simulink model "bit_sum8"  (R2014a)
settings: Solver=FixedStepDiscrete  StartTime=0.0  StopTime=10.0  RelTol=1e-3
InitFcn:
  | %% DSPBuilder Start
  | alt_dspbuilder_update_model(bdroot)
  | %% DSPBuilder End
model workspace (MAT data in the model file):
  Fs = 48000
libraries: simulink x16
settings Model: Creator=User  LastModifiedBy=User
settings DataIOCC: SaveOutput=off  SaveTime=off
settings OptimizationCC: InlineParams=on

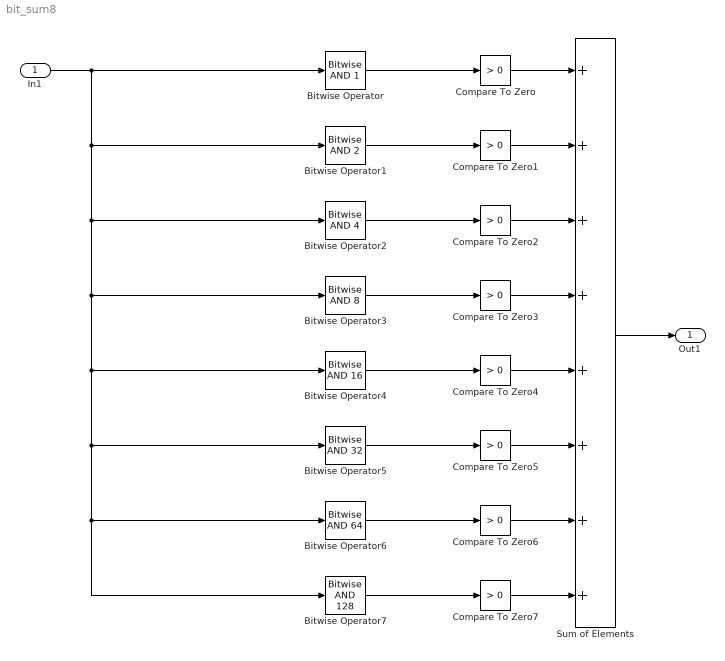
== system bit_sum8 ==
  In1 : Inport  OutDataTypeStr=uint8  PortDimensions=1
  Bitwise Operator : simulink/Logic and Bit Operations/Bitwise Operator  logicop=AND  UseBitMask=on  BitMask=1  BitMaskRealWorld=Stored Integer
  Bitwise Operator1 : simulink/Logic and Bit Operations/Bitwise Operator  logicop=AND  UseBitMask=on  BitMask=2  BitMaskRealWorld=Stored Integer
  Bitwise Operator2 : simulink/Logic and Bit Operations/Bitwise Operator  logicop=AND  UseBitMask=on  BitMask=4  BitMaskRealWorld=Stored Integer
  Bitwise Operator3 : simulink/Logic and Bit Operations/Bitwise Operator  logicop=AND  UseBitMask=on  BitMask=8  BitMaskRealWorld=Stored Integer
  Bitwise Operator4 : simulink/Logic and Bit Operations/Bitwise Operator  logicop=AND  UseBitMask=on  BitMask=16  BitMaskRealWorld=Stored Integer
  Bitwise Operator5 : simulink/Logic and Bit Operations/Bitwise Operator  logicop=AND  UseBitMask=on  BitMask=32  BitMaskRealWorld=Stored Integer
  Bitwise Operator6 : simulink/Logic and Bit Operations/Bitwise Operator  logicop=AND  UseBitMask=on  BitMask=64  BitMaskRealWorld=Stored Integer
  Bitwise Operator7 : simulink/Logic and Bit Operations/Bitwise Operator  logicop=AND  UseBitMask=on  BitMask=128  BitMaskRealWorld=Stored Integer
  Compare To Zero{,1..7} (8 alike) : simulink/Logic and Bit Operations/Compare To Zero  relop=>  OutDataTypeStr=uint8
  Sum of Elements : Sum  Inputs=++++++++  AccumDataTypeStr=uint8  OutDataTypeStr=uint8
  Out1 : Outport  OutDataTypeStr=uint8  PortDimensions=1
  wires:
  Bitwise Operator2/1 -> Compare To Zero2/1
  Bitwise Operator/1 -> Compare To Zero/1
  In1/1 -> Bitwise Operator/1, Bitwise Operator4/1, Bitwise Operator5/1, Bitwise Operator6/1, Bitwise Operator7/1, Bitwise Operator3/1, Bitwise Operator2/1, Bitwise Operator1/1
  Sum of Elements/1 -> Out1/1
  Compare To Zero6/1 -> Sum of Elements/7
  Compare To Zero4/1 -> Sum of Elements/5
  Bitwise Operator5/1 -> Compare To Zero5/1
  Compare To Zero7/1 -> Sum of Elements/8
  Bitwise Operator4/1 -> Compare To Zero4/1
  Bitwise Operator6/1 -> Compare To Zero6/1
  Bitwise Operator3/1 -> Compare To Zero3/1
  Bitwise Operator1/1 -> Compare To Zero1/1
  Compare To Zero2/1 -> Sum of Elements/3
  Bitwise Operator7/1 -> Compare To Zero7/1
  Compare To Zero3/1 -> Sum of Elements/4
  Compare To Zero/1 -> Sum of Elements/1
  Compare To Zero1/1 -> Sum of Elements/2
  Compare To Zero5/1 -> Sum of Elements/6
